simulink model "dspafsx_win32"  (Simulink 5.0)
settings: Solver=FixedStepDiscrete  StartTime=0.0  StopTime=3.928  RelTol=1e-3
PreLoadFcn:
  | load dspafxf;
libraries: simulink x3, dspwin32 x2, dspsigops x1
settings Model: CovMetricSettings=d  Creator=don  LastModifiedBy=mkhan  ExtModeTrigMode=oneshot  ExtModeArmWhenConnect=off  ExtModeAutoUpdateStatusClock=off  SaveTime=off  SaveOutput=off  LimitDataPoints=off  IntegerOverflowMsg=none  BlockReductionOpt=off  BooleanDataType=off  ZeroCrossControl=DisableAll  ProdHWWordLengths=8,32,16,32  TargetHWChar=2  TargetHWWordLengths=8,16,32,32  RTWMathFcnLibMatFile=iso_c_tmw.mat  RTWOptions="-aEnforceIntegerDowncast=1 -aFoldNonRolledExpr=1 -aInlineInvariantSignals=1 -aInlineParameters=0 -aLocalBlockOutputs=1 -aRollThreshold=2 -aRTWVerbose=1 -aForceParamTrailComments=0 -aGenerateComments=1 -aIgnoreCustomStorageClasses=1 -aIncHierarchyInIds=0 -aMaxRTWIdLen=31 -aShowEliminatedStatements=0 -aReadOnly=0 -aTargetFcnLib=\"iso_c_tmw.mat\" -aIncDataTypeInIds=0 -aPrefixModelToSubsysFcnNames=1 -aInlinedPrmAccess=\"Literals\" -aGenerateFullHeader=1 -aIsPILTarget=0 -aGenerateReport=0 -aLogVarNameModifier=\"rt_\" -aExtMode=0 -aExtModeStaticAlloc=0 -aExtModeTesting=0 -aExtModeStaticAllocSize=1000000 -aExtModeTransport=0"

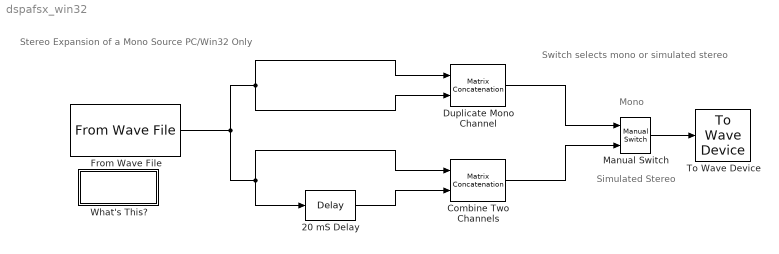
== system dspafsx_win32 ==
  note: Stereo Expansion
      | of a Mono Source
      |
      | PC/Win32 Only
  note: Switch selects mono
      | or simulated stereo
  note: Mono
  note: Simulated
      | Stereo
  20 mS Delay : dspsigops/Delay  dly_unit=Samples  delay=20e-3 * 16000  ic_detail=on  dif_ic_for_ch=off  dif_ic_for_dly=off  ic=0  reset_popup=None
  Combine Two Channels : simulink/Math Operations/Matrix Concatenation  numInports=2  catMethod=Horizontal
  Duplicate Mono Channel : simulink/Math Operations/Matrix Concatenation  numInports=2  catMethod=Horizontal
  From Wave File : dspwin32/From Wave File  FileName=dspafsx_mono  SamplesPerFrame=256  MinBufSize=256  dType=Single  bLoop=off  timesToPlay=1  restartMode=immediately after last sample  firstSampleOutput=off  lastSampleOutput=off
  Manual Switch : simulink/Signal Routing/Manual Switch  sw=0  action=0
  To Wave Device : dspwin32/To Wave Device  bufDuration=0.5  initDelay=0.1
  What's This? : Subsystem
      mask Type: Frame-Based Simulation Info
      mask Display: disp('Info')
  wires:
  20 mS Delay/1 -> Combine Two Channels/2
  Manual Switch/1 -> To Wave Device/1
  Combine Two Channels/1 -> Manual Switch/2
  From Wave File/1 -> Duplicate Mono Channel/1, Duplicate Mono Channel/2, Combine Two Channels/1, 20 mS Delay/1
  Duplicate Mono Channel/1 -> Manual Switch/1

== system dspafsx_win32/What's This? ==
  note: Stereo Signal Expansion
      |
      | For more information on acoustic effects, see:
      |     http://www.harmony-central.com
